simulink model "ziegler_nichols_2"  (R2018a)
settings: Solver=VariableStepAuto  StartTime=0.0  StopTime=10.0  RelTol=1e-3
undefined symbols (not defined in the file): Cd2_den, Cd2_num, G_den, G_num, SquareWave, T
settings Model: Creator=julio  LastModifiedBy=julio

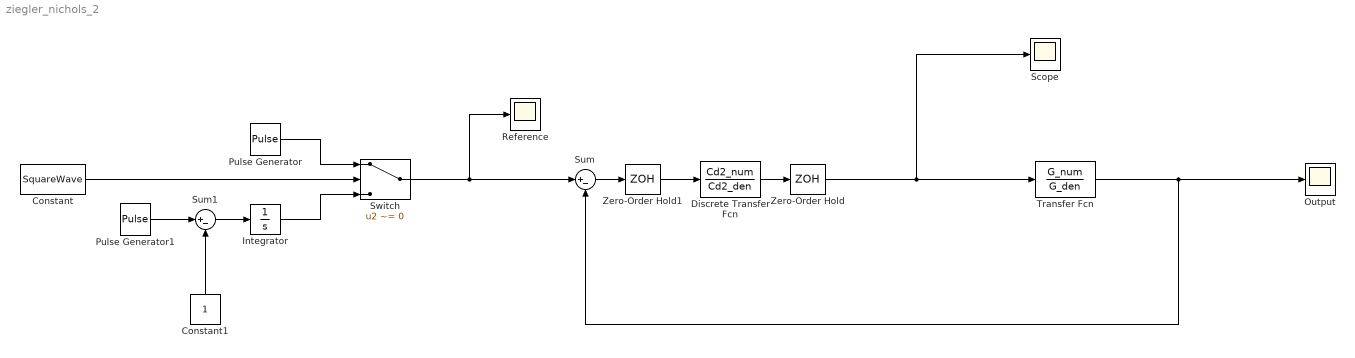
== system ziegler_nichols_2 ==
  Constant : Constant  Value=SquareWave
  Constant1 : Constant
  Discrete Transfer Fcn : DiscreteTransferFcn  Numerator=Cd2_num  Denominator=Cd2_den  SampleTime=T
  Integrator : Integrator
  Output : Scope
  Pulse Generator : DiscretePulseGenerator  PulseType=Time based  PulseWidth=50
  Pulse Generator1 : DiscretePulseGenerator  PulseType=Time based  Amplitude=2  PulseWidth=50
  Reference : Scope
  Scope : Scope
  Sum : Sum  Inputs=|+-
  Sum1 : Sum  Inputs=|+-
  Switch : Switch  Criteria=u2 ~= 0
  Transfer Fcn : TransferFcn  Numerator=G_num  Denominator=G_den
  Zero-Order Hold : ZeroOrderHold  SampleTime=T
  Zero-Order Hold1 : ZeroOrderHold  SampleTime=T
  wires:
  Discrete Transfer Fcn/1 -> Zero-Order Hold/1
  Sum/1 -> Zero-Order Hold1/1
  Transfer Fcn/1 -> Output/1, Sum/2
  Zero-Order Hold/1 -> Scope/1, Transfer Fcn/1
  Switch/1 -> Reference/1, Sum/1
  Pulse Generator/1 -> Switch/1
  Integrator/1 -> Switch/3
  Constant/1 -> Switch/2
  Sum1/1 -> Integrator/1
  Pulse Generator1/1 -> Sum1/1
  Constant1/1 -> Sum1/2
  Zero-Order Hold1/1 -> Discrete Transfer Fcn/1
